simulink model "lab_1a"  (R2020a)
settings: Solver=VariableStepAuto  StartTime=0.0  StopTime=1  RelTol=1e-3
libraries: powerlib x20
settings Model: Creator=Dhanush Wagle  LastModifiedBy=Dhanush Wagle

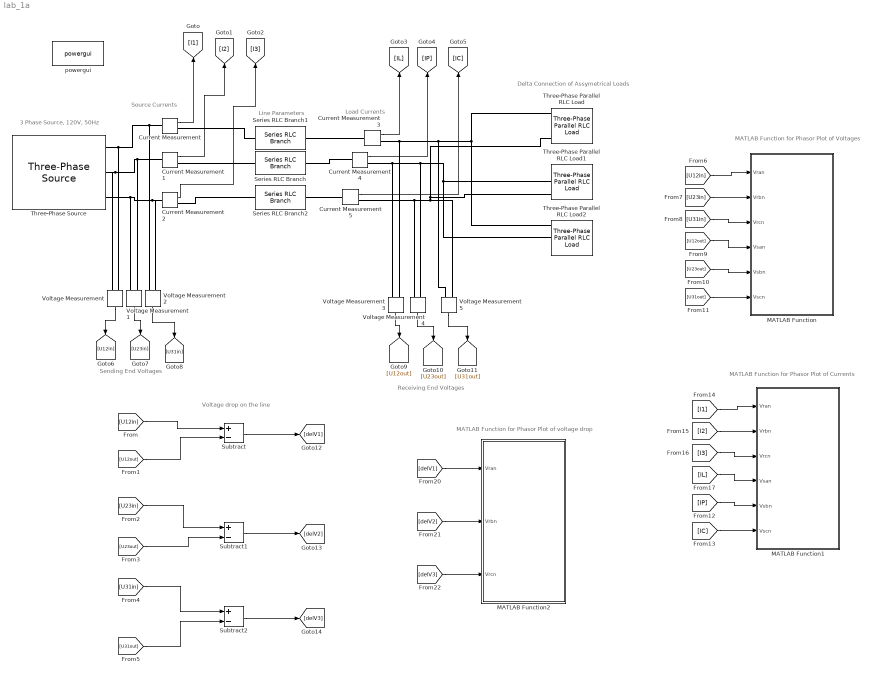
== system lab_1a ==
  note: Voltage drop on the line
  note: Delta Connection of Assymetrical Loads
  note: Receiving End Voltages
  note: Sending End Voltages
  note: Line Parameters
  note: Load Currents
  note: Source Currents
  note: 3 Phase Source, 120V, 50Hz
  note: MATLAB Function for Phasor Plot of Voltages
  note: MATLAB Function for Phasor Plot of Currents
  note: MATLAB Function for Phasor Plot of voltage drop
  Current Measurement{,1..5} (6 alike) : powerlib/Measurements/Current Measurement  PhasorSimulation=on  OutputType=Complex  PSBequivalent=0
  MATLAB Function : MATLAB Function  TreatAsAtomicUnit=on
  MATLAB Function1 : MATLAB Function  TreatAsAtomicUnit=on
  MATLAB Function2 : MATLAB Function  TreatAsAtomicUnit=on
  Series RLC Branch : powerlib/Elements/Series RLC Branch  LConnTagsString=__new0  RConnTagsString=__new0  BranchType=R  Resistance=2.12  Inductance=0  SetiL0=off  InitialCurrent=0  Capacitance=0  Setx0=off  InitialVoltage=0  Measurements=None
  Series RLC Branch1 : powerlib/Elements/Series RLC Branch  LConnTagsString=__new0  RConnTagsString=__new0  BranchType=R  Resistance=2.12  Inductance=0  SetiL0=off  InitialCurrent=0  Capacitance=0  Setx0=off  InitialVoltage=0  Measurements=None
  Series RLC Branch2 : powerlib/Elements/Series RLC Branch  LConnTagsString=__new0  RConnTagsString=__new0  BranchType=R  Resistance=2.12  Inductance=0  SetiL0=off  InitialCurrent=0  Capacitance=0  Setx0=off  InitialVoltage=0  Measurements=None
  Subtract : Sum  Inputs=+-
  Subtract1 : Sum  Inputs=+-
  Subtract2 : Sum  Inputs=+-
  Three-Phase Parallel RLC Load : powerlib/Elements/Three-Phase Parallel RLC Load  LConnTagsString=A|B|C  Configuration=Y (grounded)  NominalVoltage=120  Vabc=[1e3 1e3 1e3]  Vabcp=[1e3 1e3 1e3]  NominalFrequency=50  UnbalancedPower=off  ActivePower=0  InductivePower=235  CapacitivePower=0  Pabc=[10e3 9e3 11e3]  QLabc=[100 90 110]  QCabc=[100 90 110]  Pabcp=[10e3 9e3 11e3]  QLabcp=[100 90 110]  QCabcp=[100 90 110]  Measurements=None  LoadType=constant Z
  Three-Phase Parallel RLC Load1 : powerlib/Elements/Three-Phase Parallel RLC Load  LConnTagsString=A|B|C  Configuration=Y (grounded)  NominalVoltage=120  Vabc=[120 120 120]  Vabcp=[1e3 1e3 1e3]  NominalFrequency=50  UnbalancedPower=off  ActivePower=320  InductivePower=0  CapacitivePower=0  Pabc=[300 300 300]  QLabc=[0 0 0]  QCabc=[0 0 0]  Pabcp=[10e3 9e3 11e3]  QLabcp=[100 90 110]  QCabcp=[100 90 110]  Measurements=None  LoadType=constant Z
  Three-Phase Parallel RLC Load2 : powerlib/Elements/Three-Phase Parallel RLC Load  LConnTagsString=A|B|C  Configuration=Y (grounded)  NominalVoltage=120  Vabc=[120 120 120]  Vabcp=[1e3 1e3 1e3]  NominalFrequency=50  UnbalancedPower=off  ActivePower=0  InductivePower=0  CapacitivePower=200  Pabc=[300 300 300]  QLabc=[0 0 0]  QCabc=[0 0 0]  Pabcp=[10e3 9e3 11e3]  QLabcp=[100 90 110]  QCabcp=[100 90 110]  Measurements=None  LoadType=constant Z
  Three-Phase Source : powerlib/Electrical Sources/Three-Phase Source  InternalConnection=Yg  VoltagePhases=off  Voltage=120  PhaseAngle=0  Voltage_phases=[25e3 25e3 25e3]/sqrt(3)  PhaseAngles_phases=[0 -120 +120]  Frequency=50  NonIdealSource=on  SpecifyImpedance=off  Resistance=0.000001  Inductance=16.58e-6  ShortCircuitLevel=100e6  BaseVoltage=230  XRratio=7  BusType=swing  Pref=10e3  Qref=0  Prefabc=[10e3, 10e3, 10e3]  Qrefabc=[0, 0, 0]  Qmin=-inf  Qmax=inf
  Voltage Measurement{,1..5} (6 alike) : powerlib/Measurements/Voltage Measurement  PhasorSimulation=on  OutputType=Complex  PSBequivalent=0
  powergui : powerlib/powergui  Priority=1  SimulationMode=Phasor  SampleTime=50e-6  frequency=50  Iterations=50  frequencyindice=50  Pbase=100e6  ErrMax=1e-4  UnitsV=kV  UnitsW=MW  buscounter=0  FunctionMessages=off  echomessages=off  EnableUseOfTLC=off  CurrentSourceSwitches=off  DisableSnubberDevices=off  DisableRonSwitches=off  DisableVfSwitches=off  DisplayEquations=off  AutomaticDiscreteSolvers=off  SolverType=Tustin/Backward Euler (TBE)  Interpol=off  ExternalGateDelay=off  methode=off  Ts=100  x0status=blocks  SPID=on  SwTol=0  HookPort=off  NonlinearTolerance=1e-4  nMaxIteration=100  ContinueOnMaxIteration=off  RestoreLinks=warning  ResistiveCurrentMeasurement=off  Frange=[0:2:500]  Ylog=off  Xlog=on  ShowGrid=off  save=off  variable=ZData  structure=0  ZoomFFT=off  StartTime=0.0  cycles=1  DisplayStyle=1  fundamental=60  FreqAxis=off  MaxFrequency=1000  frequencyindicesteady=1  RmsSteady=1  display=off
  wires:
  Current Measurement/1 -> [I1]
  Current Measurement1/1 -> [I2]
  Current Measurement2/1 -> [I3]
  Current Measurement3/1 -> [IL]
  Current Measurement4/1 -> [IP]
  Current Measurement5/1 -> [IC]
  Voltage Measurement/1 -> [U12in]
  Voltage Measurement1/1 -> [U23in]
  Voltage Measurement2/1 -> [U31in]
  Voltage Measurement3/1 -> [U12out]
  Voltage Measurement4/1 -> [U23out]
  Voltage Measurement5/1 -> [U31out]
  [U12in] -> Subtract/1
  [U12out] -> Subtract/2
  Subtract/1 -> [delV1]
  [U23in] -> Subtract1/1
  [U23out] -> Subtract1/2
  Subtract1/1 -> [delV2]
  [U31in] -> Subtract2/1
  [U31out] -> Subtract2/2
  Subtract2/1 -> [delV3]
  [U12in] -> MATLAB Function/1(Vran)
  [U12out] -> MATLAB Function/4(Vsan)
  [U31in] -> MATLAB Function/3(Vrcn)
  [U23in] -> MATLAB Function/2(Vrbn)
  [U31out] -> MATLAB Function/6(Vscn)
  [U23out] -> MATLAB Function/5(Vsbn)
  [IC] -> MATLAB Function1/6(Vscn)
  [I2] -> MATLAB Function1/2(Vrbn)
  [IP] -> MATLAB Function1/5(Vsbn)
  [I3] -> MATLAB Function1/3(Vrcn)
  [I1] -> MATLAB Function1/1(Vran)
  [IL] -> MATLAB Function1/4(Vsan)
  [delV1] -> MATLAB Function2/1(Vran)
  [delV2] -> MATLAB Function2/2(Vrbn)
  [delV3] -> MATLAB Function2/3(Vrcn)
  connections:
  Three-Phase Parallel RLC Load2/LConn2 -- Current Measurement4/RConn1 -- Voltage Measurement3/LConn2 -- Voltage Measurement4/LConn1 -- Three-Phase Parallel RLC Load1/LConn2
  Three-Phase Parallel RLC Load/LConn3 -- Current Measurement5/RConn1 -- Voltage Measurement4/LConn2 -- Voltage Measurement5/LConn1 -- Three-Phase Parallel RLC Load1/LConn3
  Three-Phase Parallel RLC Load2/LConn1 -- Voltage Measurement5/LConn2 -- Voltage Measurement3/LConn1 -- Current Measurement3/RConn1 -- Three-Phase Parallel RLC Load/LConn1
  Current Measurement/LConn1 -- Voltage Measurement2/LConn2 -- Voltage Measurement/LConn1 -- Three-Phase Source/RConn1
  Current Measurement1/LConn1 -- Voltage Measurement1/LConn1 -- Voltage Measurement/LConn2 -- Three-Phase Source/RConn2
  Current Measurement2/LConn1 -- Voltage Measurement1/LConn2 -- Three-Phase Source/RConn3 -- Voltage Measurement2/LConn1
  Current Measurement/RConn1 -- Series RLC Branch1/LConn1
  Series RLC Branch/LConn1 -- Current Measurement1/RConn1
  Series RLC Branch2/LConn1 -- Current Measurement2/RConn1
  Current Measurement3/LConn1 -- Series RLC Branch1/RConn1
  Current Measurement4/LConn1 -- Series RLC Branch/RConn1
  Current Measurement5/LConn1 -- Series RLC Branch2/RConn1

== matlab function lab_1a/MATLAB Function1 ==
  data: Vran input; Vrbn input; Vrcn input; Vsan input; Vsbn input; Vscn input
function plot(Vran, Vrbn, Vrcn, Vsan, Vsbn, Vscn)

Vran = Vran;
Vrbn = Vrbn;
Vrcn = Vrcn;
Vsan = Vsan;
Vsbn = Vsbn;
Vscn = Vscn;

angle1 = angle(Vran)*ones(1,10);
angle2 = angle(Vrbn)*ones(1,10);
angle3 = angle(Vrcn)*ones(1,10);
angle4 = angle(Vsan)*ones(1,10);
angle5 = angle(Vsbn)*ones(1,10);
angle6 = angle(Vscn)*ones(1,10);

value1 = linspace(0, abs(Vran), 10);
value2 = linspace(0, abs(Vrbn), 10);
value3 = linspace(0, abs(Vrcn), 10);
value4 = linspace(0, abs(Vsan), 10);
value5 = linspace(0, abs(Vsbn), 10);
value6 = linspace(0, abs(Vscn), 10);

figure(2)
polar(angle1, value1, 'r');

hold on

polar(angle2, value2, 'y');
polar(angle3, value3, 'b');
polar(angle4, value4, 'r');
polar(angle5, value5, 'y');
polar(angle6, value6, 'b');

function set_text(V, T, ang)
text(cos(angle(V)+ang)*abs(V), sin(angle(V)+ang)*abs(V), T)
end

set_text(Vran, 'I1', 0.05)
set_text(Vrbn, 'I2', 0.05)
set_text(Vrcn, 'I3', 0.05)
set_text(Vsan, 'IL', 0.05)
set_text(Vsbn, 'IP', 0.05)
set_text(Vscn, 'IC', 0.05)

end

== matlab function lab_1a/MATLAB Function ==
  data: Vran input; Vrbn input; Vrcn input; Vsan input; Vsbn input; Vscn input
function plot(Vran, Vrbn, Vrcn, Vsan, Vsbn, Vscn)

Vran = Vran/sqrt(3);
Vrbn = Vrbn/sqrt(3);
Vrcn = Vrcn/sqrt(3);
Vsan = Vsan/sqrt(3);
Vsbn = Vsbn/sqrt(3);
Vscn = Vscn/sqrt(3);

angle1 = angle(Vran)*ones(1,10);
angle2 = angle(Vrbn)*ones(1,10);
angle3 = angle(Vrcn)*ones(1,10);
angle4 = angle(Vsan)*ones(1,10);
angle5 = angle(Vsbn)*ones(1,10);
angle6 = angle(Vscn)*ones(1,10);

value1 = linspace(0, abs(Vran), 10);
value2 = linspace(0, abs(Vrbn), 10);
value3 = linspace(0, abs(Vrcn), 10);
value4 = linspace(0, abs(Vsan), 10);
value5 = linspace(0, abs(Vsbn), 10);
value6 = linspace(0, abs(Vscn), 10);

figure(1)
polar(angle1, value1, 'r');

hold on

polar(angle2, value2, 'y');
polar(angle3, value3, 'b');
polar(angle4, value4, 'r');
polar(angle5, value5, 'y');
polar(angle6, value6, 'b');

function set_text(V, T, ang)
text(cos(angle(V)+ang)*abs(V), sin(angle(V)+ang)*abs(V), T)
end

set_text(Vran, 'U12in', 0.05)
set_text(Vrbn, 'U23in', 0.05)
set_text(Vrcn, 'U31in', 0.05)
set_text(Vsan, 'U12out', 0.05)
set_text(Vsbn, 'U23out', 0.05)
set_text(Vscn, 'U31out', 0.05)

end

== matlab function lab_1a/MATLAB Function2 ==
  data: Vran input; Vrbn input; Vrcn input
function plot(Vran, Vrbn, Vrcn)

Vran = Vran/sqrt(3);
Vrbn = Vrbn/sqrt(3);
Vrcn = Vrcn/sqrt(3);


angle1 = angle(Vran)*ones(1,10);
angle2 = angle(Vrbn)*ones(1,10);
angle3 = angle(Vrcn)*ones(1,10);


value1 = linspace(0, abs(Vran), 10);
value2 = linspace(0, abs(Vrbn), 10);
value3 = linspace(0, abs(Vrcn), 10);

figure(3)
polar(angle1, value1, 'r');

hold on

polar(angle2, value2, 'y');
polar(angle3, value3, 'b');

function set_text(V, T, ang)
text(cos(angle(V)+ang)*abs(V), sin(angle(V)+ang)*abs(V), T)
end

set_text(Vran, 'del_U1', 0.05)
set_text(Vrbn, 'del_U2', 0.05)
set_text(Vrcn, 'del_U3', 0.05)


end
